simulink subsystem "ControlAdapter"  (R2025a)
settings: Solver=VariableStepAuto  StartTime=0.0  StopTime=10.0  RelTol=1e-3
settings Model: Creator=Глеб  LastModifiedBy=Глеб

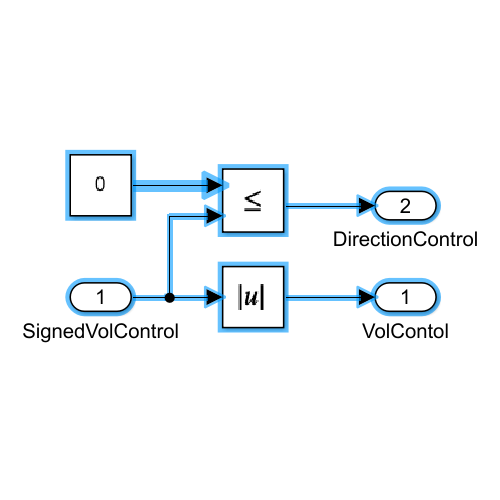
[thumbnail: Simulink's stored preview of the top-level diagram]
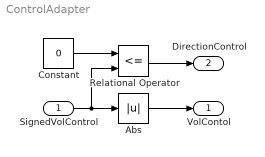
== system ControlAdapter ==
  SignedVolControl : Inport
  Abs : Abs  SaturateOnIntegerOverflow=off
  Constant : Constant  Value=0
  Relational Operator : RelationalOperator  Operator=<=  OutDataTypeStr=boolean  RndMeth=Simplest  InputSameDT=off
  VolContol : Outport
  DirectionControl : Outport  Port=2  OutDataTypeStr=boolean
  wires:
  SignedVolControl/1 -> Relational Operator/2, Abs/1
  Abs/1 -> VolContol/1
  Relational Operator/1 -> DirectionControl/1
  Constant/1 -> Relational Operator/1
